simulink model "Aula12-7.4"  (R2023a)
settings: Solver=VariableStepAuto  StartTime=0.0  StopTime=10.0  RelTol=1e-3
libraries: simulink x2
settings Model: Creator=a2320606  LastModifiedBy=a2320606

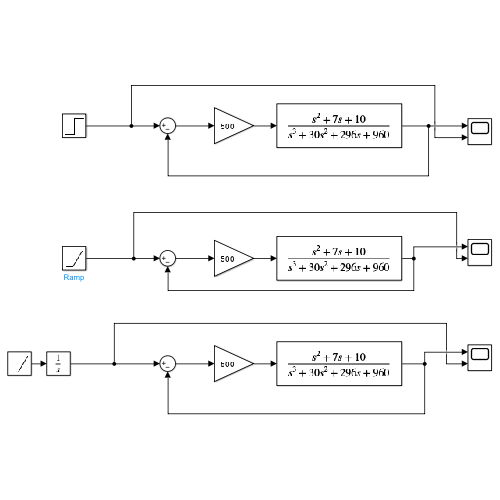
[thumbnail: Simulink's stored preview of the top-level diagram]
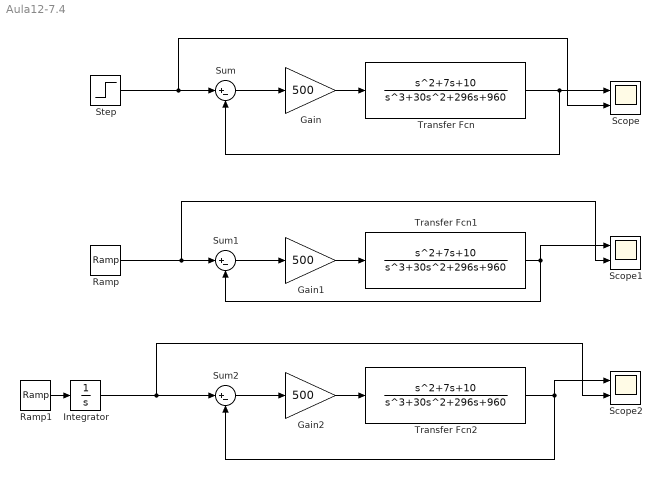
== system Aula12-7.4 ==
  Gain : Gain  Gain=500
  Gain1 : Gain  Gain=500
  Gain2 : Gain  Gain=500
  Integrator : Integrator
  Ramp : simulink/Sources/Ramp  slope=1  start=0  InitialOutput=0
  Ramp1 : simulink/Sources/Ramp  slope=1  start=0  InitialOutput=0
  Scope : Scope  NumInputPorts=2
  Scope1 : Scope  NumInputPorts=2
  Scope2 : Scope  NumInputPorts=2
  Step : Step  SampleTime=0
  Sum : Sum  Inputs=|+-
  Sum1 : Sum  Inputs=|+-
  Sum2 : Sum  Inputs=|+-
  Transfer Fcn : TransferFcn  Numerator=[1 7 10]  Denominator=[1 30 296 960]
  Transfer Fcn1 : TransferFcn  Numerator=[1 7 10]  Denominator=[1 30 296 960]
  Transfer Fcn2 : TransferFcn  Numerator=[1 7 10]  Denominator=[1 30 296 960]
  wires:
  Transfer Fcn/1 -> Scope/1, Sum/2
  Sum/1 -> Gain/1
  Gain/1 -> Transfer Fcn/1
  Sum1/1 -> Gain1/1
  Transfer Fcn1/1 -> Scope1/1, Sum1/2
  Gain1/1 -> Transfer Fcn1/1
  Step/1 -> Scope/2, Sum/1
  Ramp/1 -> Sum1/1, Scope1/2
  Gain2/1 -> Transfer Fcn2/1
  Sum2/1 -> Gain2/1
  Transfer Fcn2/1 -> Scope2/1, Sum2/2
  Integrator/1 -> Scope2/2, Sum2/1
  Ramp1/1 -> Integrator/1
